simulink model "controlador"  (R2023b)
settings: Solver=ode23t  StartTime=0.0  StopTime=60  MaxStep=1e-3  RelTol=1e-3
values from neighbouring files (symbols this model uses):
  AL = double(subs(A_par))    [ANTImodeloMATEMATICOFINAL.m]
  BL = double(subs(B_par))    [ANTImodeloMATEMATICOFINAL.m]
  Blo = 8.18575752786119e-06    (= 8.18575752786e-06)    [ANTImodeloMATEMATICOFINAL.m]
  Bmo = 2.02156082362446e-07    (= 2.02156082362e-07)    [ANTImodeloMATEMATICOFINAL.m]
  CL = double(subs(C_par))    [ANTImodeloMATEMATICOFINAL.m]
  DL = double(subs(D_par))    [ANTImodeloMATEMATICOFINAL.m]
  do = 0.06862-0.021    (= 0.04762)    [ANTImodeloMATEMATICOFINAL.m]
  go = 9.81    [ANTImodeloMATEMATICOFINAL.m]
  Jlo = 0.00100697016255642    (= 0.00100697016256)    [ANTImodeloMATEMATICOFINAL.m]
  Jmo = 2.08549279330578e-07    (= 2.08549279331e-07)    [ANTImodeloMATEMATICOFINAL.m]
  Kes = K(:,1:n)    [ANTImodeloMATEMATICOFINAL.m]
  Ki = -K(:,n+1:end)    [ANTImodeloMATEMATICOFINAL.m]
  Kio = 0.00119530882984502    (= 0.00119530882985)    [ANTImodeloMATEMATICOFINAL.m]
  Kvo = 0.0035694528924319    (= 0.00356945289243)    [ANTImodeloMATEMATICOFINAL.m]
  Lo = 0.667669785204658    (= 0.667669785205)    [ANTImodeloMATEMATICOFINAL.m]
  mo = 0.17244    [ANTImodeloMATEMATICOFINAL.m]
  no = 120    [ANTImodeloMATEMATICOFINAL.m]
  Ro = 5.15610211779038    (= 5.15610211779)    [ANTImodeloMATEMATICOFINAL.m]
  Tm = 0.03    [ANTImodeloMATEMATICOFINAL.m]
  Vin0 = Ro*X10    (= 0)    [ANTImodeloMATEMATICOFINAL.m]
  X10 = 0    [ANTImodeloMATEMATICOFINAL.m]
  X20 = 0    [ANTImodeloMATEMATICOFINAL.m]
  X30 = 0    [ANTImodeloMATEMATICOFINAL.m]
undefined symbols (not defined in the file or in its folder): Ac_2, Bc_2, Cc_2, Dc_2, L, magnitude, sys_d2
libraries: cstblocks x6, slpidlib x4, simulink x4
(part 2 of 2)

== system controlador/Seg. Estados Desacop-/Subsystem5 ==
  In1 : Inport
  Abs : Abs  SaturateOnIntegerOverflow=off
  Clock : Clock
  Clock1 : Clock
  Integrator{3..6} (4 alike) : Integrator
  Power : Math  Operator=magnitude^2  SignedPower=on
  Product : Product
  Product1 : Product
  IAE : Outport  VectorParamsAs1DForOutWhenUnconnected=off
  ITAE : Outport  Port=2  VectorParamsAs1DForOutWhenUnconnected=off
  ISE : Outport  Port=3  VectorParamsAs1DForOutWhenUnconnected=off
  ITSE : Outport  Port=4  VectorParamsAs1DForOutWhenUnconnected=off
  wires:
  Clock/1 -> Product/2
  Power/1 -> Integrator5/1, Product1/1
  Product1/1 -> Integrator6/1
  Abs/1 -> Product/1, Integrator3/1
  Clock1/1 -> Product1/2
  Product/1 -> Integrator4/1
  Integrator3/1 -> IAE/1
  Integrator6/1 -> ITSE/1
  Integrator4/1 -> ITAE/1
  In1/1 -> Power/1, Abs/1
  Integrator5/1 -> ISE/1

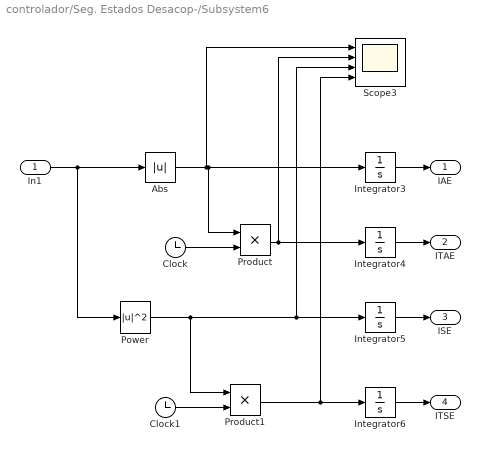
== system controlador/Seg. Estados Desacop-/Subsystem6 ==
  In1 : Inport
  Abs : Abs  SaturateOnIntegerOverflow=off
  Clock : Clock
  Clock1 : Clock
  Integrator{3..6} (4 alike) : Integrator
  Power : Math  Operator=magnitude^2  SignedPower=on
  Product : Product
  Product1 : Product
  Scope3 : Scope  NumInputPorts=4
  IAE : Outport  VectorParamsAs1DForOutWhenUnconnected=off
  ITAE : Outport  Port=2  VectorParamsAs1DForOutWhenUnconnected=off
  ISE : Outport  Port=3  VectorParamsAs1DForOutWhenUnconnected=off
  ITSE : Outport  Port=4  VectorParamsAs1DForOutWhenUnconnected=off
  wires:
  Integrator5/1 -> ISE/1
  In1/1 -> Abs/1, Power/1
  Integrator4/1 -> ITAE/1
  Integrator6/1 -> ITSE/1
  Integrator3/1 -> IAE/1
  Product/1 -> Scope3/2, Integrator4/1
  Clock1/1 -> Product1/2
  Abs/1 -> Scope3/1, Integrator3/1, Product/1
  Product1/1 -> Scope3/4, Integrator6/1
  Power/1 -> Product1/1, Scope3/3, Integrator5/1
  Clock/1 -> Product/2

== matlab function controlador/Estados Discreto/Subsystem1/MATLAB Function ==
  data: x input; PWM input; dx output; parametros input
function dx = fcn(x,PWM,parametros)

%ESTADOS
x1 = x(1);
x2 = x(2);

%Parametros
R = parametros(1);
L = parametros(2);
Ki = parametros(3);
Kv = parametros(4);
Jm = parametros(5);
Jl = parametros(6);
Bm = parametros(7);
Bl = parametros(8);
n = parametros(9);
g = parametros(10);
d = parametros(11);
m = parametros(12);

%EXPRESIONES
f1 = x2; %d0l/dt = Wl
f2= ((Ki*(((7*PWM/100)-(Kv*x2*n)/R))*n)-x2*(Bm*n^2+Bl)-(m*g*d*sin(x1)))/(Jl+Jm*n^2);

dx = [f1; f2];

== matlab function controlador/PID Cascada Discreto/Subsystem1/MATLAB Function ==
  data: x input; PWM input; dx output; parametros input
function dx = fcn(x,PWM,parametros)

%ESTADOS
x1 = x(1);
x2 = x(2);
x3 = x(3);

%Parametros
R = parametros(1);
L = parametros(2);
Ki = parametros(3);
Kv = parametros(4);
Jm = parametros(5);
Jl = parametros(6);
Bm = parametros(7);
Bl = parametros(8);
n = parametros(9);
g = parametros(10);
d = parametros(11);
m = parametros(12);

%EXPRESIONES
% Jt = Jm*n^2 +Jl;
% f1 = (1/L)*(((7*PWM)/100) - R*x1 - Kv*x2*n);
% f2 = (1/Jt)*(Ki*x1*n - (Bm*n^2 + Bl)*x2 - m*g*d*sin(x3));
% f3 = x2;

% MODELO 2 ESTADOS I TL WL  SALIDA TL WL
f1 = (((7*PWM)/100)-Kv*x3*n-R*x1)/(L); %di/dt
f2 = x3; %d0l/dt = Wl
f3 = ((Ki*x1*n)-x3*(Bm*n^2+Bl)-(m*g*d*sin(x2)))/(Jl+Jm*n^2);  %dwl/dt 

dx = [f1; f2; f3];

== matlab function controlador/PID 1 DOF /Subsystem/MATLAB Function ==
  data: x input; PWM input; dx output; parametros input
function dx = fcn(x,PWM,parametros)

%ESTADOS
x1 = x(1);
x2 = x(2);
x3 = x(3);

%Parametros
R = parametros(1);
L = parametros(2);
Ki = parametros(3);
Kv = parametros(4);
Jm = parametros(5);
Jl = parametros(6);
Bm = parametros(7);
Bl = parametros(8);
n = parametros(9);
g = parametros(10);
d = parametros(11);
m = parametros(12);

%EXPRESIONES
% Jt = Jm*n^2 +Jl;
% f1 = (1/L)*(((7*PWM)/100) - R*x1 - Kv*x2*n);
% f2 = (1/Jt)*(Ki*x1*n - (Bm*n^2 + Bl)*x2 - m*g*d*sin(x3));
% f3 = x2;

% MODELO 2 ESTADOS I TL WL  SALIDA TL WL
f1 = (((7*PWM)/100)-Kv*x3*n-R*x1)/(L); %di/dt
f2 = x3; %d0l/dt = Wl
f3 = ((Ki*x1*n)-x3*(Bm*n^2+Bl)-(m*g*d*sin(x2)))/(Jl+Jm*n^2);  %dwl/dt 

dx = [f1; f2; f3];

== matlab function controlador/PID 1 DOF Discreto/Subsystem/MATLAB Function ==
  data: x input; PWM input; dx output; parametros input
function dx = fcn(x,PWM,parametros)

%ESTADOS
x1 = x(1);
x2 = x(2);
x3 = x(3);

%Parametros
R = parametros(1);
L = parametros(2);
Ki = parametros(3);
Kv = parametros(4);
Jm = parametros(5);
Jl = parametros(6);
Bm = parametros(7);
Bl = parametros(8);
n = parametros(9);
g = parametros(10);
d = parametros(11);
m = parametros(12);
Cm = 0.005;

if x3 > 0
    Ft = Bm*sign(x3) - Cm*x3;
elseif x3 <0
        Ft = Bm*sign(x3) + Cm*x3;
else
    Ft = 0;
end



if abs(PWM)<20
    x3 = 0;
end



% MODELO 2 ESTADOS I TL WL  SALIDA TL WL
f1 = (((7*PWM)/100)-Kv*x3*n-R*x1)/(L); %di/dt
f2 = x3; %d0l/dt = Wl
f3 = ((Ki*x1*n)-x3*(Bm*n^2+Bl)-(m*g*d*sin(x2)) - Ft)/(Jl+Jm*n^2);  %dwl/dt 

if abs(PWM)<20
    f3= 0;
end

dx = [f1; f2; f3];



% function dx = fcn(x,PWM,parametros)
% 
% %ESTADOS
% x1 = x(1);
% x2 = x(2);
% x3 = x(3);
% 
% %Parametros
% R = parametros(1);
% L = parametros(2);
% Ki = parametros(3);
% Kv = parametros(4);
% Jm = parametros(5);
% Jl = parametros(6);
% Bm = parametros(7);
% Bl = parametros(8);
% n = parametros(9);
% g = parametros(10);
% d = parametros(11);
% m = parametros(12);
% V = 3.94;
% % Incluir los parametros añadidos
% % Incluir la diiferencia de PWM que se debe aplciar al motor para que este
% % cambie de posicion EN LAZO ABIERTO
% difPWM = 30;
% % Incluir la velocidad minima que puede mantener el motor
% velMinima = 0.05;
% 
% if abs(PWM)<30
%     x3 = 0;
% end
% 
% Fs = ((difPWM*V/100)/R)*(Ki+Kv); % Friccion estatica
% Fc = Fs/8; % Friccion de Coulumb
% % Determinar la friccion TOTAL que se aplica al modelo
% % Torque externo
% Tex = - m*g*d*sin(x2) + (Ki+Kv)*x1;
% % Si la velocidad es menor a la velocidad minima entonces se aplica
% % FRICCION ESTATICA
% if(abs(x3) <= velMinima)
% if(abs(Tex) <= (Fs))
% % la friccion es igual al torque externo
% Ft = -Tex ;
% else
% % la friccion es igual a la suma de las fricciones
% Ft = -(Fs)*sign(Tex);
% end
% % Si la velocidad es mayor a la velocidad minima entonces se aplica
% % FRICCION COULUMB (unicamente)
% else
% Ft = -Fc*sign(x3);
% end
% 
% 
% 
% 
% 
% 
% % MODELO 2 ESTADOS I TL WL  SALIDA TL WL
% % MODELO 2 ESTADOS I TL WL  SALIDA TL WL
% f1 = (((7*PWM)/100)-Kv*x3*n-R*x1)/(L); %di/dt
% f2 = x3; %d0l/dt = Wl
% f3 = ((Ki*x1*n)-x3*(Bm*n^2+Bl)-(m*g*d*sin(x2)) - Ft)/(Jl+Jm*n^2);  %dwl/dt 
% 
% if abs(PWM)<30
%     f3 = 0;
% end
% 
% dx = [f1; f2; f3];

== matlab function controlador/Estados Discreto/MATLAB Function ==
  data: Sp input; us output; X_est input; Con_ini input; Con_out output
function [us,Con_out] = fcn(Sp,X_est,Con_ini)

umax = 100;
umin = -100;
kaw = zeros(1);
CL = [1, 0]
Ki = [13.038404810405284];
Kes = [8.39272964861829,6.19627625077861];

Vk_1 = Con_ini(1);
dif_act = Con_ini(2);

Tm = 0.03;
Kid = Ki*Tm;

Pv = CL*X_est;
en = Sp - Pv;
Vk = en + Vk_1 + kaw*dif_act;
un = Kid*Vk - Kes*X_est;
us = un;

Vk_1 = Vk;

if un>umax
    us = umax;
end
if un<umin
    us = umin;
end

dif_act = us - un;
Con_out = [Vk_1; dif_act];

== matlab function controlador/PID 1 DOF Discreto/MATLAB Function1 ==
  data: Sp input; us output; Pv input; Con_ini input; Con_out output
% function [us, Con_out] = fcn(Sp, Pv, Con_ini)
%  
% en_1 = Con_ini(1);
% en_2 = Con_ini(2);
% un_1 = Con_ini(3);
% un_2 = Con_ini(4);
% difact = Con_ini(5);
% umin = -100;
% umax = 100;
% kaw = 0.1; 
%  
% en = Sp - Pv;
% un = 52.346730287862997*en - 99.613623826288730*en_1 + 48.365148241217845*en_2 + 1.742509213223832*un_1 - 0.742509213223832*un_2 + kaw*difact;
%  
% us = un;
%  
% if un < umin 
%     us = umin;
% end
% if un > umax 
%     us = umax;
% end
%  
% en_2 = en_1;
% en_1 = en;
% un_2 = un_1;
% un_1 = un;
% difact = us - un;
%          
% Con_out = [en_1; en_2; un_1; un_2; difact];

function [us, Con_out] = fcn(Sp, Pv, Con_ini)

en_1 = Con_ini(1);
I_error_1 = Con_ini(2);
difact = Con_ini(3);
Ad_1 = Con_ini(4);

umin = -100;
umax = 100;

Kp = 12.194801852041582;
Ki = 1.836264365827931;
Kd = 58.215749090323079;
N = 0.135321750384943;
kaw=0.1; 


en = Sp - Pv;
Ap = Kp*en;
Ad = Kd*(en-en_1) + N*Ad_1;
I_error = en + I_error_1 + kaw*difact;
Ai = Ki*I_error;
un = Ap + Ai + Ad;
us = un;

if un < umin 
    us = umin;
end
if un > umax 
    us = umax;
end

en_1 = en;
I_error_1 = I_error;
difact = us - un;
Ad_1 = Ad;
      
Con_out = [en_1; I_error_1; difact; Ad_1];

== matlab function controlador/PID 1 DOF Discreto/MATLAB Function2 ==
  data: Sp input; us output; Pv input; Con_ini input; Con_out output
function [us, Con_out] = fcn(Sp, Pv, Con_ini)

en_1 = Con_ini(1);
I_error_1 = Con_ini(2);
difact = Con_ini(3);
Ad_1 = Con_ini(4);
us_1 = Con_ini(5);

umin = -100;
umax = 100;

Kp = 12.194801852041582;
Ki = 1.836264365827931;
Kd = 58.215749090323079;
N = 0.135321750384943;
kaw = 0.1; 

en = Sp - Pv;

if abs(en) > abs(Sp*0.065)
    Ap = Kp*en;
    Ad = Kd*(en-en_1) + N*Ad_1;
    I_error = en + I_error_1 + kaw*difact;
    Ai = Ki*I_error;
    un = Ap + Ai + Ad;
    us = un;

    if un < umin 
        us = umin;
    end
    if un > umax 
        us = umax;
    end

    en_1 = en;
    I_error_1 = I_error;
    difact = us - un;
    Ad_1 = Ad;
    us_1 = us;

else
    us = us_1; % Asignar el último valor de us
end

Con_out = [en_1; I_error_1; difact; Ad_1; us_1];

% 
% function [us, Con_out] = fcn(Sp, Pv, Con_ini)
% 
% en_1 = Con_ini(1);
% I_error_1 = Con_ini(2);
% difact = Con_ini(3);
% Ad_1 = Con_ini(4);
% us_1 = Con_ini(5);
% 
% umin = -100;
% umax = 100;
% 
% Kp = 12.194801852041582;
% Ki = 1.836264365827931;
% Kd = 58.215749090323079;
% N = 0.135321750384943;
% kaw = 0.1; 
% 
% en = Sp - Pv;
% 
%     Ap = Kp*en;
%     Ad = Kd*(en-en_1) + N*Ad_1;
%     I_error = en + I_error_1 + kaw*difact;
%     Ai = Ki*I_error;
%     un = Ap + Ai + Ad;
%     us = un;
% 
%     if un < umin 
%         us = umin;
%     end
%     if un > umax 
%         us = umax;
%     end
% 
%     en_1 = en;
%     I_error_1 = I_error;
%     difact = us - un;
%     Ad_1 = Ad;
%     us_1 = us;
% 
% 
% 
% Con_out = [en_1; I_error_1; difact; Ad_1; us_1];

== matlab function controlador/PID 2 DOF/Subsystem/MATLAB Function ==
  data: x input; PWM input; dx output; parametros input
function dx = fcn(x,PWM,parametros)

%ESTADOS
x1 = x(1);
x2 = x(2);
x3 = x(3);

%Parametros
R = parametros(1);
L = parametros(2);
Ki = parametros(3);
Kv = parametros(4);
Jm = parametros(5);
Jl = parametros(6);
Bm = parametros(7);
Bl = parametros(8);
n = parametros(9);
g = parametros(10);
d = parametros(11);
m = parametros(12);

%EXPRESIONES
% Jt = Jm*n^2 +Jl;
% f1 = (1/L)*(((7*PWM)/100) - R*x1 - Kv*x2*n);
% f2 = (1/Jt)*(Ki*x1*n - (Bm*n^2 + Bl)*x2 - m*g*d*sin(x3));
% f3 = x2;

% MODELO 2 ESTADOS I TL WL  SALIDA TL WL
f1 = (((7*PWM)/100)-Kv*x3*n-R*x1)/(L); %di/dt
f2 = x3; %d0l/dt = Wl
f3 = ((Ki*x1*n)-x3*(Bm*n^2+Bl)-(m*g*d*sin(x2)))/(Jl+Jm*n^2);  %dwl/dt 

dx = [f1; f2; f3];

== matlab function controlador/PID 2 DOF Discreto/MATLAB Function ==
  data: Sp input; us output; Pv input; Con_ini input; Con_out output
% function [us, Con_out] = fcn(Sp, Pv, Con_ini)
%  
% en_1 = Con_ini(1);
% u1_1 = Con_ini(2);
% Pv_1 = Con_ini(3);
% u2_1 = Con_ini(4);
% difact = Con_ini(5);
% umin = -100;
% umax = 100;
% kaw = 0.01; 
%  
% en = Sp - Pv;
% u1 = 0.153958966653420*en_1 + u1_1 + kaw*difact;
% u2 = 22.177058343736231*Pv - 21.573923642220816*(Pv_1) + 0.732201155629244*u2_1;
% un = u1-u2;
% us = un;
%  
% if un < umin 
%     us = umin;
% end
% if un > umax 
%     us = umax;
% end
%  
% en_1 = en;
% u1_1 = u1;
% Pv_1 = Pv;
% u2_1 = u2;
% difact = us - un;
%          
% Con_out = [en_1; u1_1; Pv_1;u2_1; difact];

function [us, Con_out] = fcn(Sp, Pv, Con_ini)

en_1 = Con_ini(1);
yn_1 = Con_ini(2);
I_error_1 = Con_ini(3);
difact = Con_ini(4);
Ad_1 = Con_ini(5);
Ad1_ = Con_ini(6);

umin = -100;
umax = 100;

Kp = -3.357670445385118;
Ki = 3.822951239710286;
Kd = 32.464560395668343;
N = 0.782109908780621;
Kpd = 0.285776886757601;
Kdp = 3.408050560944484;
N1 = 0.997168715666942;
Ka= 0.1; 

en =  Sp - Pv;
Ap = Kp*en;
Ad = Kd*(en-en_1) + N*Ad1_;
I_error = en + I_error_1 + Ka*difact;
Ai = Ki*I_error;
U1 = Ap + Ai + Ad;

Ap1 = Kpd * Pv;
Ad1 = Kdp * (Pv - yn_1) + N1*Ad_1;
U2 = Ap1 + Ad1;

Uc = U1 - U2;
us = Uc;


if Uc < umin 
    us = umin;
end
if Uc > umax 
    us = umax;
end

en_1 = en;
yn_1 = Pv;
I_error_1 = I_error;
difact = us - Uc;
Ad_1 = Ad1;
Ad1_ = Ad;
      
Con_out = [en_1; yn_1; I_error_1; difact; Ad_1; Ad1_];

== matlab function controlador/PID 2 DOF Discreto/Subsystem/MATLAB Function ==
  data: x input; PWM input; dx output; parametros input
function dx = fcn(x,PWM,parametros)

%ESTADOS
x1 = x(1);
x2 = x(2);
x3 = x(3);

%Parametros
R = parametros(1);
L = parametros(2);
Ki = parametros(3);
Kv = parametros(4);
Jm = parametros(5);
Jl = parametros(6);
Bm = parametros(7);
Bl = parametros(8);
n = parametros(9);
g = parametros(10);
d = parametros(11);
m = parametros(12);

%EXPRESIONES
% Jt = Jm*n^2 +Jl;
% f1 = (1/L)*(((7*PWM)/100) - R*x1 - Kv*x2*n);
% f2 = (1/Jt)*(Ki*x1*n - (Bm*n^2 + Bl)*x2 - m*g*d*sin(x3));
% f3 = x2;

% MODELO 2 ESTADOS I TL WL  SALIDA TL WL
f1 = (((7*PWM)/100)-Kv*x3*n-R*x1)/(L); %di/dt
f2 = x3; %d0l/dt = Wl
f3 = ((Ki*x1*n)-x3*(Bm*n^2+Bl)-(m*g*d*sin(x2)))/(Jl+Jm*n^2);  %dwl/dt 

dx = [f1; f2; f3];

== matlab function controlador/PID 2 DOF Discreto/MATLAB Function1 ==
  data: Sp input; us output; Pv input; Con_ini input; Con_out output
% function [us, Con_out] = fcn(Sp, Pv, Con_ini)
%  
% en_1 = Con_ini(1);
% u1_1 = Con_ini(2);
% Pv_1 = Con_ini(3);
% u2_1 = Con_ini(4);
% difact = Con_ini(5);
% umin = -100;
% umax = 100;
% kaw = 0.01; 
%  
% en = Sp - Pv;
% u1 = 0.153958966653420*en_1 + u1_1 + kaw*difact;
% u2 = 22.177058343736231*Pv - 21.573923642220816*(Pv_1) + 0.732201155629244*u2_1;
% un = u1-u2;
% us = un;
%  
% if un < umin 
%     us = umin;
% end
% if un > umax 
%     us = umax;
% end
%  
% en_1 = en;
% u1_1 = u1;
% Pv_1 = Pv;
% u2_1 = u2;
% difact = us - un;
%          
% Con_out = [en_1; u1_1; Pv_1;u2_1; difact];

function [us, Con_out] = fcn(Sp, Pv, Con_ini)

en_1 = Con_ini(1);
yn_1 = Con_ini(2);
I_error_1 = Con_ini(3);
difact = Con_ini(4);
Ad_1 = Con_ini(5);
Ad1_ = Con_ini(6);

umin = -100;
umax = 100;

% Kp = 0.01357670445385118;
% Ki = 1.822951239710286;
% Kd = 10.464560395668343;
% N = 0.782109908780621;
% Kpd = 1.285776886757601;
% Kdp = 13.408050560944484;
% N1 = 0.997168715666942;
% Ka= 0.1;

Kp = -3.357670445385118;
Ki = 3.822951239710286;
Kd = 32.464560395668343;
N = 0.782109908780621;
Kpd = 0.285776886757601;
Kdp = 3.408050560944484;
N1 = 0.997168715666942;
Ka= 0.1; 

en =  Sp - Pv;
Ap = Kp*en;
Ad = Kd*(en-en_1) + N*Ad1_;
I_error = en + I_error_1 + Ka*difact;
Ai = Ki*I_error;
U1 = Ap + Ai + Ad;

Ap1 = Kpd * Pv;
Ad1 = Kdp * (Pv - yn_1) + N1*Ad_1;
U2 = Ap1 + Ad1;

Uc = U1 - U2;
us = Uc;


if Uc < umin 
    us = umin;
end
if Uc > umax 
    us = umax;
end

en_1 = en;
yn_1 = Pv;
I_error_1 = I_error;
difact = us - Uc;
Ad_1 = Ad1;
Ad1_ = Ad;
      
Con_out = [en_1; yn_1; I_error_1; difact; Ad_1; Ad1_];

== matlab function controlador/Estados Discreto/MATLAB Function1 ==
  data: Sp input; us output; X_est input; Con_ini input; Con_out output
function [us,Con_out] = fcn(Sp,X_est,Con_ini)

umax = 100;
umin = -100;
kaw = zeros(1);
CL = [1, 0]
Ki = [13.038404810405284];
Kes = [8.39272964861829,6.19627625077861];

Vk_1 = Con_ini(1);
dif_act = Con_ini(2);

Tm = 0.03;
Kid = Ki*Tm;

Pv = CL*X_est;
en = Sp - Pv;
Vk = en + Vk_1 + kaw*dif_act;
un = Kid*Vk - Kes*X_est;
us = un;

Vk_1 = Vk;

if un>umax
    us = umax;
end
if un<umin
    us = umin;
end

dif_act = us - un;
Con_out = [Vk_1; dif_act];

== matlab function controlador/PID Cascada Discreto/MATLAB Function1 ==
  data: Sp input; u2 output; Pv input; Pv1 input; Con_ini input; Con_out output
function [u2,Con_out] = fcn(Sp,Pv,Pv1,Con_ini)

en_1 = Con_ini(1);
u1_1 = Con_ini(2);
en2_1 = Con_ini(3);
u2_1 = Con_ini(4);

en = Sp - Pv;
u1 = 0.439531738224972*en + 0.093106585918219*en_1+1*u1_1;
en_1 = en;
u1_1 = u1;

u1min = -40;
u1max = 40;

if u1_1 < u1min 
    u1 = u1min;
end
if u1_1 > u1max 
    u1 = u1max;
end

en2 = u1 - Pv1;
u2 = 0*en2 + 93.138459952280698*en2_1+1*u2_1;
en2_1 = en2;
u2_1 = u2;

u2min = -100;
u2max = 100;

if u2_1 < u2min 
    u2 = u2min;
end
if u2_1 > u2max 
    u2 = u2max;
end

Con_out = [en_1; u1_1; en2_1; u2_1];

== matlab function controlador/PID Cascada Discreto/MATLAB Function ==
  data: Sp input; u2 output; Pv input; Pv1 input; Con_ini input; Con_out output
function [u2,Con_out] = fcn(Sp,Pv,Pv1,Con_ini)

en_1 = Con_ini(1);
u1_1 = Con_ini(2);
en2_1 = Con_ini(3);
u2_1 = Con_ini(4);

en = Sp - Pv;
u1 = 0.439531738224972*en + 0.093106585918219*en_1+1*u1_1;
en_1 = en;
u1_1 = u1;

u1min = -40;
u1max = 40;

if u1_1 < u1min 
    u1 = u1min;
end
if u1_1 > u1max 
    u1 = u1max;
end

en2 = u1 - Pv1;
u2 = 0*en2 + 93.138459952280698*en2_1+1*u2_1;
en2_1 = en2;
u2_1 = u2;

u2min = -100;
u2max = 100;

if u2_1 < u2min 
    u2 = u2min;
end
if u2_1 > u2max 
    u2 = u2max;
end

Con_out = [en_1; u1_1; en2_1; u2_1];

== matlab function controlador/Seg. Estados Desacop-/Subsystem2/MATLAB Function ==
  data: x input; PWM input; dx output; parametros input
function dx = fcn(x,PWM,parametros)

%ESTADOS
x1 = x(1);
x2 = x(2);
x3 = x(3);

%Parametros
R = parametros(1);
L = parametros(2);
Ki = parametros(3);
Kv = parametros(4);
Jm = parametros(5);
Jl = parametros(6);
Bm = parametros(7);
Bl = parametros(8);
n = parametros(9);
g = parametros(10);
d = parametros(11);
m = parametros(12);

%EXPRESIONES
% Jt = Jm*n^2 +Jl;
% f1 = (1/L)*(((7*PWM)/100) - R*x1 - Kv*x2*n);
% f2 = (1/Jt)*(Ki*x1*n - (Bm*n^2 + Bl)*x2 - m*g*d*sin(x3));
% f3 = x2;

% MODELO 2 ESTADOS I TL WL  SALIDA TL WL
f1 = (((7*PWM)/100)-Kv*x3*n-R*x1)/(L); %di/dt
f2 = x3; %d0l/dt = Wl
f3 = ((Ki*x1*n)-x3*(Bm*n^2+Bl)-(m*g*d*sin(x2)))/(Jl+Jm*n^2);  %dwl/dt 

dx = [f1; f2; f3];

== matlab function controlador/Seg. Estados 2DOF Discreto/Subsystem2/MATLAB Function ==
  data: x input; PWM input; dx output; parametros input
function dx = fcn(x,PWM,parametros)

%ESTADOS
x1 = x(1);
x2 = x(2);
x3 = x(3);

%Parametros
R = parametros(1);
L = parametros(2);
Ki = parametros(3);
Kv = parametros(4);
Jm = parametros(5);
Jl = parametros(6);
Bm = parametros(7);
Bl = parametros(8);
n = parametros(9);
g = parametros(10);
d = parametros(11);
m = parametros(12);

%EXPRESIONES
% Jt = Jm*n^2 +Jl;
% f1 = (1/L)*(((7*PWM)/100) - R*x1 - Kv*x2*n);
% f2 = (1/Jt)*(Ki*x1*n - (Bm*n^2 + Bl)*x2 - m*g*d*sin(x3));
% f3 = x2;

% MODELO 2 ESTADOS I TL WL  SALIDA TL WL
f1 = (((7*PWM)/100)-Kv*x3*n-R*x1)/(L); %di/dt
f2 = x3; %d0l/dt = Wl
f3 = ((Ki*x1*n)-x3*(Bm*n^2+Bl)-(m*g*d*sin(x2)))/(Jl+Jm*n^2);  %dwl/dt 

dx = [f1; f2; f3];

== matlab function controlador/Seg. Estados 2DOF Discreto/MATLAB Function2 ==
  data: Sp input; u output; Pv input; Con_ini input; Con_out output
function [u,Con_out] = fcn(Sp,Pv,Con_ini)
Gc = [0.945300903756753	0.00617052631399497	-0.0133691286278173	0.0136794859742906
0.000157886661775223	0.999905507978029	0.00299590182719107	7.43870391104292e-07
0.104240134112312	-0.0598706998014357	0.997004271824335	0.000740282375445457
0	0	0	1];
Hc = [2.07115790289755e-05	-2.04869120105457e-05
5.59520825196690e-10	4.48576312528050e-06
7.43871227858539e-07	-8.63703141685189e-07
0.00300000000000000	-0.00300000000000000];
Cc = [-102.796775094683	18.8434497806398	-37.6657368965828	44.7213595499950];
Dc = [0	0];

u1max = 100;
u1min = -100;

Ka = zeros(4,1);

xk = Con_ini(1:4);  %n+r
Du = Con_ini(5:5);  %p

u = Cc*xk + Dc*[Sp;Pv];
xk_1 = Gc*xk + Hc*[Sp;Pv] - Ka*Du;

% Hsp = [0.000536712016934462,0.000277774040110453;0.00110188262899529,-0.000214997449972678;5.70600160926339e-05,0.000178431372314633;0.000111261745162715,-0.000748573895925450;0.0600000000000000,0;0,0.0600000000000000];
% Hpv = [0.528743127428489,-0.0440381830752178;0.441160175174069,0.0425524022491926;-0.00772595368821204,0.204727393044363;-0.0185719938075179,0.0357506408044768;-0.0600000000000000,0;0,-0.0600000000000000];
% u = Cc*xk;
% xk_1 = Gc*xk + Hsp*Sp + Hpv*Pv - Ka*Du;

u1s = u(1);

if u(1)>=u1max
    u1s = u1max;
end
if u(1)<=u1min
    u1s = u1min;
end



%% Salida
ut = u1s;
Dunew = u - ut;
Con_out = [xk_1; Dunew];

== matlab function controlador/Seg. Estados 2DOF Discreto/MATLAB Function1 ==
  data: Sp input; u output; Pv input; Con_ini input; Con_out output
function [u,Con_out] = fcn(Sp,Pv,Con_ini)
Gc = [0.883560462392427	-4.13249708388486e-12	-0.00487572121212935	0.135443000110772	-0.00479641932613010
-0.000588434369415533	0.644036421083143	0.00829798816152157	-4.57027036271401e-05	0.00866807794337489
-0.00487572121200123	1.30651084000254e-14	0.577392998520158	-0.000392434304393785	1.35422668727884
0	0	0	1	0
0	0	0	0	1];
Hc = [0.00138236824312267	-3.37592528540001e-05	0.00971261372273124	0.00632660435715394
-3.16147125121532e-07	6.26926980241918e-05	0.000624297068749436	-0.0109217038882698
-2.76212064284266e-06	0.0147757234577708	0.00518371001609480	0.00771884768968612
0.0200000000000000	0	-0.0200000000000000	0
0	0.0200000000000000	0	-0.0200000000000000];
Cc = [2.60000000006463	3.87499999993181	-0.750000000024670	1.79999999984347	9.96447369061571e-11
-4.30872282297656e-11	-2.25000000000000	0.499999999999999	1.04354552776798e-10	1.64313007644523e-14
-2.80000000007810	-1.93749999996589	-11.1249999999877	-0.899999999768644	43.9999999999502];
Dc = [0	0	0	0
0	0	0	0
0	0	0	0];

u1max = 10;
u1min = -10;
u2max = 10;
u2min = -10;
u3max = 10;
u3min = -10;

Ka = zeros(5,3);

xk = Con_ini(1:5);  %n+r
Du = Con_ini(6:8);  %p

u = Cc*xk + Dc*[Sp;Pv];
xk_1 = Gc*xk + Hc*[Sp;Pv] - Ka*Du;

% Hsp = [0.000536712016934462,0.000277774040110453;0.00110188262899529,-0.000214997449972678;5.70600160926339e-05,0.000178431372314633;0.000111261745162715,-0.000748573895925450;0.0600000000000000,0;0,0.0600000000000000];
% Hpv = [0.528743127428489,-0.0440381830752178;0.441160175174069,0.0425524022491926;-0.00772595368821204,0.204727393044363;-0.0185719938075179,0.0357506408044768;-0.0600000000000000,0;0,-0.0600000000000000];
% u = Cc*xk;
% xk_1 = Gc*xk + Hsp*Sp + Hpv*Pv - Ka*Du;

u1s = u(1);
u2s = u(2);
u3s = u(3);

if u(1)>=u1max
    u1s = u1max;
end
if u(1)<=u1min
    u1s = u1min;
end

if u(2)>=u2max
    u2s = u2max;
end
if u(2)<=u2min
    u2s = u2min;
end

if u(3)>=u3max
    u3s = u3max;
end
if u(3)<=u3min
    u3s = u3min;
end

%% Salida
ut = [u1s;u2s;u3s];
Dunew = u - ut;
Con_out = [xk_1; Dunew];

== matlab function controlador/PID Cascada/Subsystem1/MATLAB Function ==
  data: x input; PWM input; dx output; parametros input
function dx = fcn(x,PWM,parametros)

%ESTADOS
x1 = x(1);
x2 = x(2);
x3 = x(3);

%Parametros
R = parametros(1);
L = parametros(2);
Ki = parametros(3);
Kv = parametros(4);
Jm = parametros(5);
Jl = parametros(6);
Bm = parametros(7);
Bl = parametros(8);
n = parametros(9);
g = parametros(10);
d = parametros(11);
m = parametros(12);

%EXPRESIONES
% Jt = Jm*n^2 +Jl;
% f1 = (1/L)*(((7*PWM)/100) - R*x1 - Kv*x2*n);
% f2 = (1/Jt)*(Ki*x1*n - (Bm*n^2 + Bl)*x2 - m*g*d*sin(x3));
% f3 = x2;

% MODELO 2 ESTADOS I TL WL  SALIDA TL WL
f1 = (((7*PWM)/100)-Kv*x3*n-R*x1)/(L); %di/dt
f2 = x3; %d0l/dt = Wl
f3 = ((Ki*x1*n)-x3*(Bm*n^2+Bl)-(m*g*d*sin(x2)))/(Jl+Jm*n^2);  %dwl/dt 

dx = [f1; f2; f3];

== matlab function controlador/Seg. Estados/Subsystem2/MATLAB Function ==
  data: x input; PWM input; dx output; parametros input
function dx = fcn(x,PWM,parametros)

%ESTADOS
x1 = x(1);
x2 = x(2);

%Parametros
R = parametros(1);
L = parametros(2);
Ki = parametros(3);
Kv = parametros(4);
Jm = parametros(5);
Jl = parametros(6);
Bm = parametros(7);
Bl = parametros(8);
n = parametros(9);
g = parametros(10);
d = parametros(11);
m = parametros(12);

%EXPRESIONES
f1 = x2; %d0l/dt = Wl
f2= ((Ki*(((7*PWM/100)-(Kv*x2*n)/R))*n)-x2*(Bm*n^2+Bl)-(m*g*d*sin(x1)))/(Jl+Jm*n^2);

dx = [f1; f2];
